simulink model "clik_inverse_z"  (R2022b)
settings: Solver=VariableStepAuto  StartTime=0.0  StopTime=10.0  RelTol=1e-3
undefined symbols (not defined in the file or in its folder): DiscIntNeverNeededParam, q0, Tc
settings Model: Creator=josh7  LastModifiedBy=brigh
settings SolverCC: AlgebraicLoopSolver=TrustRegion
settings DebuggingCC: UnconnectedInputMsg=warning  UnconnectedOutputMsg=warning  UnconnectedLineMsg=warning  SFMachineParentedDataDiag=warning  ArithmeticOperatorsInVariantConditions=warning
settings ModelReferenceCC: EnableRefExpFcnMdlSchedulingChecks=on
settings SFSimCC: CustomCodeUndefinedFunction=UseInterfaceOnly
settings RTWCC: DLArmComputeVersion=19.05

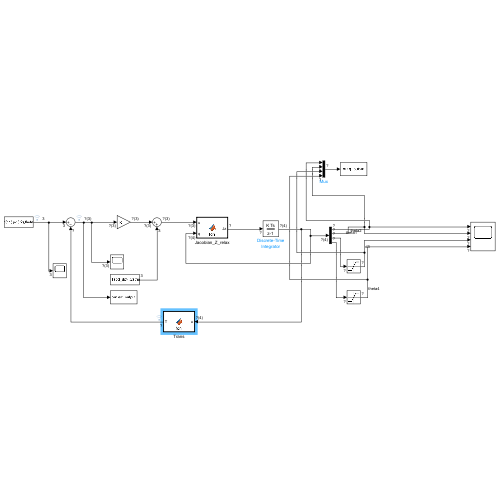
[thumbnail: Simulink's stored preview of the top-level diagram]
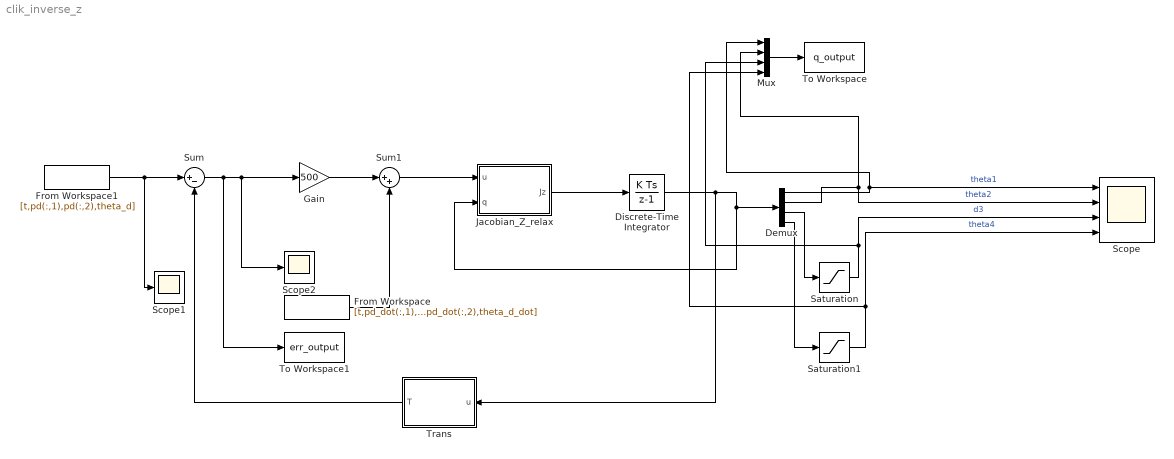
== system clik_inverse_z ==
  Demux : Demux
  Discrete-Time Integrator : DiscreteIntegrator  InitialCondition=q0  SampleTime=Tc  ICPrevOutput=DiscIntNeverNeededParam  ICPrevScaledInput=DiscIntNeverNeededParam
  From Workspace : FromWorkspace  VariableName=[t,pd_dot(:,1),pd_dot(:,2),theta_d_dot]  SampleTime=Tc
  From Workspace1 : FromWorkspace  VariableName=[t,pd(:,1),pd(:,2),theta_d]  SampleTime=Tc
  Gain : Gain  Gain=500
  "Jacobian_Z_relax " : MATLAB Function  TreatAsAtomicUnit=on
  Mux : Mux
  Saturation : Saturate  UpperLimit=1  LowerLimit=0.25
  Saturation1 : Saturate  UpperLimit=4.713  LowerLimit=-4.713
  Scope : Scope  NumInputPorts=4
  Scope1 : Scope
  Scope2 : Scope
  Sum : Sum  Inputs=|+-
  Sum1 : Sum  Inputs=|++
  To Workspace : ToWorkspace  VariableName=q_output  SampleTime=-1
  To Workspace1 : ToWorkspace  VariableName=err_output  SampleTime=-1
  Trans : MATLAB Function  TreatAsAtomicUnit=on
  wires:
  Gain/1 -> Sum1/1
  Trans/1(T) -> Sum/2
  "Jacobian_Z_relax "/1(Jz) -> Discrete-Time Integrator/1
  Discrete-Time Integrator/1 -> Trans/1(u), "Jacobian_Z_relax "/2(q), Demux/1
  Sum1/1 -> "Jacobian_Z_relax "/1(u)
  From Workspace/1 -> Sum1/2
  From Workspace1/1 -> Scope1/1, Sum/1
  Sum/1 -> To Workspace1/1, Scope2/1, Gain/1
  Demux/1 -> Mux/1, Scope/1  "theta1"
  Demux/2 -> Mux/2, Scope/2  "theta2"
  Demux/3 -> Saturation/1
  Saturation/1 -> Scope/3, Mux/3  "d3"
  Demux/4 -> Saturation1/1
  Saturation1/1 -> Scope/4, Mux/4  "theta4"
  Mux/1 -> To Workspace/1

== matlab function clik_inverse_z/Jacobian_Z_relax  ==
  data: u input; Jz output; q input
function Jz = fcn(u,q)

a1 = 0.5;
a2 = 0.5;
d3 = q(3);

theta1 = q(1);
theta12 = theta1+q(2);

cos1 = cos(theta1);
sin1 = sin(theta1);
cos12 = cos(theta12);
sin12 = sin(theta12);

k = 10;

J = [-a2*sin12-a1*sin1 -a2*sin12 0 0; a2*cos12+a1*cos1 a2*cos12 0 0; 1 1 0 1];

jp = pinv(J);

ki = jp * u;

c = eye(4) - (jp * J);

p=[0.4;-0.7;0.5;1];


qd=[-(2*(sin(theta12)/2 + sin(q(1))/2)*(cos(theta12)/2 + cos(q(1))/2 - p(1,:)) - 2*(cos(theta12)/2 + cos(q(1))/2)*(sin(theta12)/2 + sin(q(1))/2 + p(2,:)))/(2*((cos(theta12)/2 + cos(q(1))/2 - p(1,:))^2 + (sin(theta12)/2 + sin(q(1))/2 + p(2,:))^2 + (q(3) - p(3,:))^2)^(1/2)),  -(sin(theta12)*(cos(theta12)/2 + cos(q(1))/2 - p(1,:)) - cos(theta12)*(sin(theta12)/2 + sin(q(1))/2 + p(2,:)))/(2*((cos(theta12)/2 + cos(q(1))/2 - p(1,:))^2 + (sin(theta12)/2 + sin(q(1))/2 + p(2,:))^2 + (q(3) - p(3,:))^2)^(1/2)),  (2*q(3) - 1)/(2*((cos(theta12)/2 + cos(q(1))/2 - p(1,:))^2 + (sin(theta12)/2 + sin(q(1))/2 + p(2,:))^2 + (q(3) - p(3,:))^2)^(1/2)), 0];


g =k* qd.';

Jz = ki + (c * g);
end

== matlab function clik_inverse_z/Trans ==
  data: u input; T output
function T = fcn(u)

a1=0.5;
a2 = 0.5;

b = u(1) + u(2);
cos1 = cos(u(1));
sin1 = sin(u(1));
cos12 = cos(b);
sin12 = sin(b);


T= [a2*cos12+a1*cos1; a2*sin12+a1*sin1; u(1)+u(2)+u(4)];
